simulink model "Nomoto2"  (R2015b)
settings: Solver=ode45  StartTime=tstart  StopTime=tstop  RelTol=1e-3
values from neighbouring files (symbols this model uses):
  delta_c = dc_list(i)    [NonLinearAnalysis.m]    (also in Run_Delta_R_Sim.m = d_list(i); analyse_lin_dynamics.m = deg2rad(delta_list(i)); analyse_ulin_dynamics kopi.m = deg2rad(delta); analyse_ulin_dynamics.m = deg2rad(delta_list(i)))
  tsamp = 10    [NonLinearAnalysis.m]    (also in analyse_lin_dynamics.m; analyse_steadystate.m; analyse_ulin_dynamics kopi.m; analyse_ulin_dynamics.m)
  x = lsqcurvefit(F4, x0, t, r,[20 0],[500 0.15],OPT)    [analyse_lin_dynamics.m]    (also in analyse_ulin_dynamics kopi.m = lsqcurvefit(F8, x0, t, r,[],[],OPT); analyse_ulin_dynamics.m = lsqcurvefit(F8, x0, t, r,[0 0],[400 1],OPT); curvefitting.m = lsqcurvefit(F, x0, t, r); run.m = lsqcurvefit(F_4, x0, t, r))
settings Model: ExtModeAutoUpdateStatusClock=off  Creator=christh  LastModifiedBy=Erik
settings DataIOCC: SaveFormat=Array  SignalLoggingSaveFormat=ModelDataLogs
settings OptimizationCC: ExpressionDepthLimit=2147483647  InitFltsAndDblsToZero=on
settings DebuggingCC: UnderspecifiedInitializationDetection=Classic  MergeDetectMultiDrivingBlocksExec=none  SolverPrmCheckMsg=warning  FcnCallInpInsideContextMsg=UseLocalSettings  StateNameClashWarn=warning
settings HardwareCC: ProdBitPerPointer=32  ProdLargestAtomicFloat=None  ProdIntDivRoundTo=Undefined  ProdEndianess=Unspecified  ProdWordSize=32  ProdHWDeviceType=32-bit Generic
settings GRTTargetCC: GeneratePreprocessorConditionals=Disable all  CombineOutputUpdateFcns=off  GRTInterface=on
settings ConfigComp: CovModelRefEnable=Off

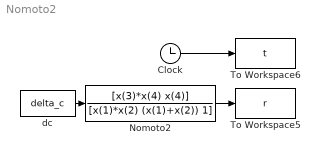
== system Nomoto2 ==
  Clock : Clock
  Nomoto2 : TransferFcn  Numerator=[x(3)*x(4) x(4)]  Denominator=[x(1)*x(2) (x(1)+x(2)) 1]
  To Workspace5 : ToWorkspace  VariableName=r  SampleTime=tsamp
  To Workspace6 : ToWorkspace  VariableName=t  SampleTime=tsamp
  dc : Constant  Value=delta_c
  wires:
  Clock/1 -> To Workspace6/1
  dc/1 -> Nomoto2/1
  Nomoto2/1 -> To Workspace5/1
